simulink model "UpperLimb_TrajectoryGenerator"  (R2024b)
settings: Solver=VariableStepAuto  StartTime=0.0  StopTime=10.0  RelTol=1e-3
settings Model: Creator=jakub  LastModifiedBy=jakub

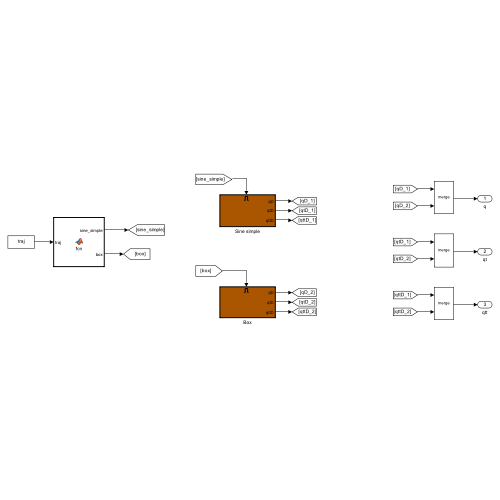
[thumbnail: Simulink's stored preview of the top-level diagram]
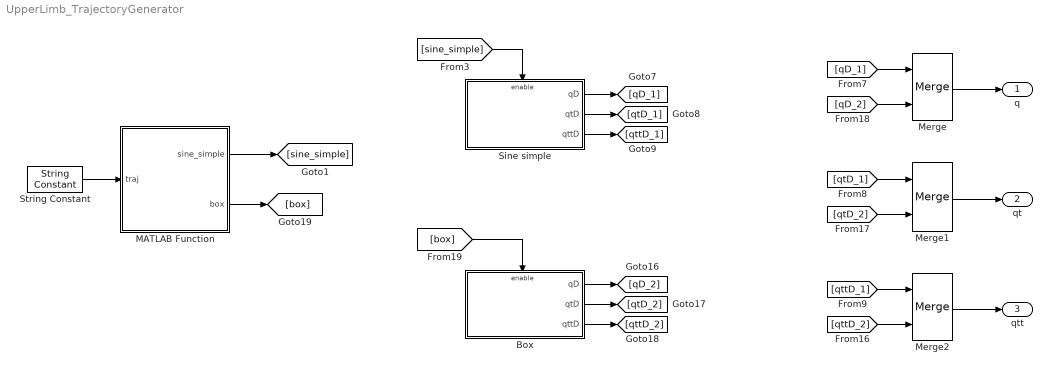
== system UpperLimb_TrajectoryGenerator ==
  Box : Subsystem
  MATLAB Function : MATLAB Function  TreatAsAtomicUnit=on
  Merge : Merge
  Merge1 : Merge
  Merge2 : Merge
  Sine simple : Subsystem  TreatAsAtomicUnit=on
  String Constant : StringConstant  String=traj
  q : Outport  OutDataTypeStr=double  Unit=rad  PortDimensions=[2 1]  SampleTime=0
  qt : Outport  Port=2  OutDataTypeStr=double  Unit=rad/sec  PortDimensions=[2 1]  SampleTime=0
  qtt : Outport  Port=3  OutDataTypeStr=double  Unit=rad/s^2  PortDimensions=[2 1]  SampleTime=0
  wires:
  Box/3(qttD) -> [qttD_2]
  [box] -> Box/Enable
  Sine simple/2(qtD) -> [qtD_1]
  Merge/1 -> q/1
  Sine simple/3(qttD) -> [qttD_1]
  Sine simple/1(qD) -> [qD_1]
  String Constant/1 -> MATLAB Function/1(traj)
  [qD_2] -> Merge/2
  Merge1/1 -> qt/1
  Merge2/1 -> qtt/1
  MATLAB Function/1(sine_simple) -> [sine_simple]
  Box/1(qD) -> [qD_2]
  MATLAB Function/2(box) -> [box]
  Box/2(qtD) -> [qtD_2]
  [sine_simple] -> Sine simple/Enable
  [qD_1] -> Merge/1
  [qtD_1] -> Merge1/1
  [qtD_2] -> Merge1/2
  [qttD_1] -> Merge2/1
  [qttD_2] -> Merge2/2

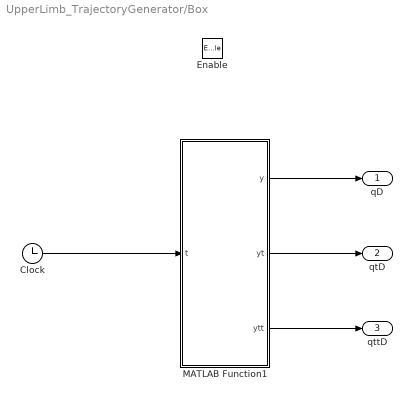
== system UpperLimb_TrajectoryGenerator/Box ==
  Enable : EnablePort
  Clock : Clock
  MATLAB Function1 : MATLAB Function  TreatAsAtomicUnit=on
  qD : Outport  OutDataTypeStr=double  Unit=rad  PortDimensions=[2 1]
  qtD : Outport  Port=2  OutDataTypeStr=double  Unit=rad/s  PortDimensions=[2 1]
  qttD : Outport  Port=3  OutDataTypeStr=double  Unit=rad/s^2  PortDimensions=[2 1]
  wires:
  Clock/1 -> MATLAB Function1/1(t)
  MATLAB Function1/1(y) -> qD/1
  MATLAB Function1/2(yt) -> qtD/1
  MATLAB Function1/3(ytt) -> qttD/1

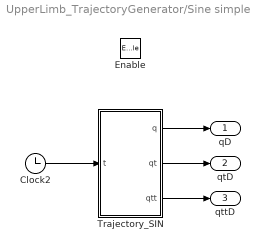
== system UpperLimb_TrajectoryGenerator/Sine simple ==
  Enable : EnablePort
  Clock2 : Clock
  Trajectory_SIN : MATLAB Function  TreatAsAtomicUnit=on
  qD : Outport
  qtD : Outport  Port=2
  qttD : Outport  Port=3
  wires:
  Clock2/1 -> Trajectory_SIN/1(t)
  Trajectory_SIN/1(q) -> qD/1
  Trajectory_SIN/2(qt) -> qtD/1
  Trajectory_SIN/3(qtt) -> qttD/1

== matlab function UpperLimb_TrajectoryGenerator/MATLAB Function ==
  data: traj input string; sine_simple output double size=1; box output double size=1
function [sine_simple, box] = fcn(traj)

sine_simple = 0;
box = 0;

switch traj
    case "sine_simple"
        sine_simple = 1;

    case "box"
        box = 1;
end

== matlab function UpperLimb_TrajectoryGenerator/Sine simple/Trajectory_SIN ==
  data: t input; q output; qt output; qtt output
function [q, qt, qtt] = fcn(t)

% Trajectory 1
    % f1 = 0.5;
    % f2 = 0.5;

% Trajectory 3 - BICB, BRACH injury 90%
    f1 = 1.3;
    f2 = 1.3;  

% % REV #3 - response 1Hz
%     f1 = 1;
%     f2 = 1;
% % REV #3 - response 2Hz
%     f1 = 2;
%     f2 = 2;


om1 = 2*pi*f1;
om2 = 2*pi*f2;
psi = -pi/2;


A01 = -pi/4;
A02 = pi/4;
A1 = 0.5*pi/4;
A2 = 0.7*2/4*pi;


fi12 = A01 + A1*sin(om1*t + psi);
fi12t = om1*A1*cos(om1*t + psi);
fi12tt = -om1^2*A1*sin(om1*t + psi);


fi13 = A02 + A2*sin(om2*t + psi);
fi13t = om2*A2*cos(om2*t + psi);
fi13tt = -om2^2*A2*sin(om2*t + psi);

q = [fi12;fi13];
qt = [fi12t;fi13t];
qtt = [fi12tt; fi13tt];

== matlab function UpperLimb_TrajectoryGenerator/Box/MATLAB Function1 ==
  data: t input double size=1; y output double size=[2 1]; yt output double size=[2 1]; ytt output double size=[2 1]
function [y,yt,ytt] = fcn(t)

stred12 = (-0.1*pi/2 - 0.9*pi/2)/2;
stred13 = (0.1*pi/2 + 0.7*pi/2)/2;

% Trajectory 2
f = 1;

om = 2*pi*f;
psi = pi/2;

A2 = 0.4*pi/2;
A3 = 0.25*pi/2;

fi12 = stred12 + A2*sin(om*t+psi);
fi12t = A2*om*cos(om*t+psi);
fi12tt = -A2*om^2*sin(om*t+psi);

fi13 = stred13 - A3*sin(om*t+psi);
fi13t = - A3*om*cos(om*t+psi);
fi13tt = + A3*om^2*sin(om*t+psi);



y = [fi12;fi13];
yt = [fi12t; fi13t];
ytt = [fi12tt; fi13tt];
